simulink model "PID_testing"  (R2023b)
settings: Solver=VariableStepAuto  StartTime=0.0  StopTime=10.0  RelTol=1e-3
values from neighbouring files (symbols this model uses):
  B = 1.36e-6    (= 1.36e-06)    [Admittance_code.m]    (also in motor_model_state_space.m = [0 ; 0 ; 1/L])
  J = 1.62e-6    (= 1.62e-06)    [Admittance_code.m]    (also in motor_model_state_space.m = 1e-06)
  Ke = 0.011    [Admittance_code.m]    (also in motor_model_state_space.m)
  Kt = 0.011    [Admittance_code.m]    (also in motor_model_state_space.m)
  L = 0.58E-3    (= 0.00058)    [Admittance_code.m]    (also in motor_model_state_space.m)
  R = 1.17    [Admittance_code.m]    (also in motor_model_state_space.m)
libraries: slpidlib x1
settings Model: Creator=sayeh  LastModifiedBy=sayeholoumi

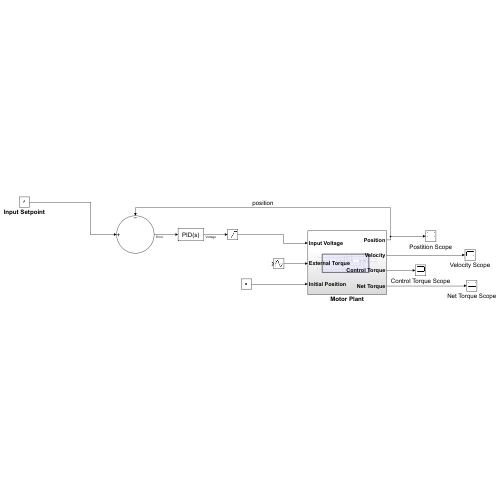
[thumbnail: Simulink's stored preview of the top-level diagram]
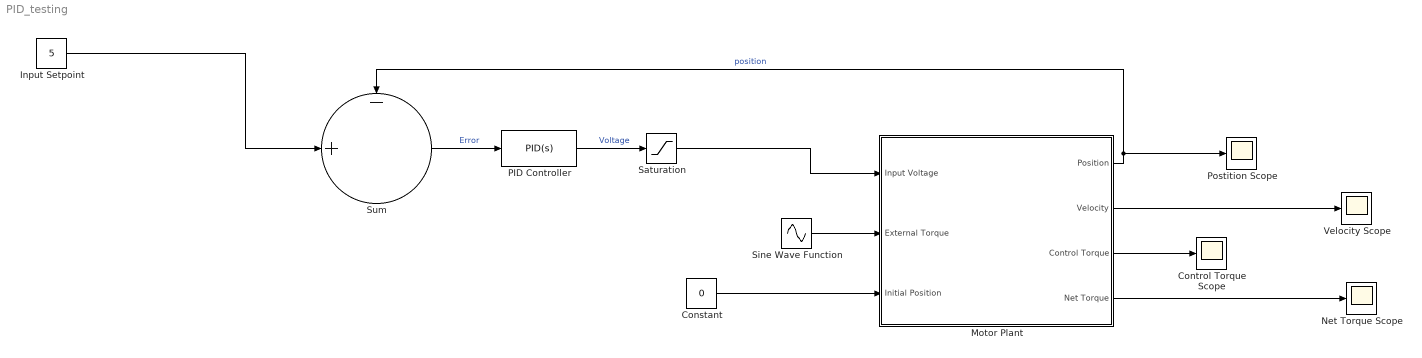
== system PID_testing ==
  Constant : Constant  Value=0
  Control Torque Scope : Scope
  Input Setpoint : Constant  Value=5
  Motor Plant : Subsystem
  Net Torque Scope : Scope
  PID Controller : slpidlib/PID Controller  Controller=PID  Form=Parallel  TimeDomain=Continuous-time  UseExternalTs=off  SampleTime=-1  IntegratorMethod=Forward Euler  FilterMethod=Forward Euler  ControllerParametersSource=internal  P=2  I=10  UseKiTs=off  D=0.0208927627785181  N=1000  UseFilter=on  TunerSelectOption=Transfer Function Based (PID Tuner App)  InitialConditionSource=internal  InitialConditionForIntegrator=0  InitialConditionForFilter=0  DifferentiatorICPrevScaledInput=0  ExternalReset=none  TrackingMode=off  Kt=1  LimitOutput=off  SatLimitsSource=internal  UpperSaturationLimit=inf  LowerSaturationLimit=-inf  LinearizeAsGain=on  AntiWindupMode=none  Kb=1  LimitIntegrator=off  UpperIntegratorSaturationLimit=inf  LowerIntegratorSaturationLimit=-inf  POutMin=[]  POutMax=[]  IOutMin=[]  IOutMax=[]  DOutMin=[]  DOutMax=[]  NOutMin=[]  NOutMax=[]  SumOutMin=[]  SumOutMax=[]  SaturationOutMin=[]  SaturationOutMax=[]  PParamMin=[]  PParamMax=[]  IParamMin=[]  IParamMax=[]  DParamMin=[]  DParamMax=[]  NParamMin=[]  NParamMax=[]  KbParamMin=[]  KbParamMax=[]  KtParamMin=[]  KtParamMax=[]  KbOutMin=[]  KbOutMax=[]  KtOutMin=[]  KtOutMax=[]  IntegratorOutMin=[]  IntegratorOutMax=[]  FilterOutMin=[]  FilterOutMax=[]  SumI1OutMin=[]  SumI1OutMax=[]  SumI2OutMin=[]  SumI2OutMax=[]  SumI3OutMin=[]  SumI3OutMax=[]  SumI4OutMin=[]  SumI4OutMax=[]  SumDOutMin=[]  SumDOutMax=[]  DifferentiatorOutMin=[]  DifferentiatorOutMax=[]  FilterDiffOutCoefMin=[]  FilterDiffOutCoefMax=[]  ReciprocalOutMin=[]  ReciprocalOutMax=[]  SumDenOutMin=[]  SumDenOutMax=[]  SumNumOutMin=[]  SumNumOutMax=[]  DivideOutMin=[]  DivideOutMax=[]  UdiffTsProdOutMin=[]  UdiffTsProdOutMax=[]  NTsProdOutMin=[]  NTsProdOutMax=[]  UintegralTsProdOutMin=[]  UintegralTsProdOutMax=[]  UngainTsProdOutMin=[]  UngainTsProdOutMax=[]  ClampingZeroOutDataTypeStr=Inherit: Inherit via back propagation  ClampingZeroOutMin=[]  ClampingZeroOutMax=[]  FilterDenConstantOutDataTypeStr=Inherit: Inherit via back propagation  FilterDenConstantOutMin=[]  FilterDenConstantOutMax=[]  PCopyOutDataTypeStr=Inherit: Inherit via back propagation  PCopyOutMin=[]  PCopyOutMax=[]  NCopyOutDataTypeStr=Inherit: Inherit via back propagation  NCopyOutMin=[]  NCopyOutMax=[]  IntegratorContinuousStateAttributes=''  IntegratorStateMustResolveToSignalObject=off  IntegratorRTWStateStorageClass=Auto  FilterContinuousStateAttributes=''  FilterStateMustResolveToSignalObject=off  FilterRTWStateStorageClass=Auto  ParallelPVariant=InternalParameters  IdealPVariant=Disabled  IVariant=InternalParameters  DVariant=InternalParameters  IntegratorVariant=Continuous  SatVariant=Disabled  AWVariant=Passthrough  PCopyVariant=Disabled  TRVariant=Disabled  FdbkBlocksVariant=Forward  IdealPFdbkVariant=Disabled  SatFdbkVariant=Disabled  DerivativeFilterVariant=ContFilter  NVariant=InternalParameters  NCopyVariant=Disabled  FilterICVariant=InternalICsFilter  IntegratorICVariant=InternalICs  ExternalResetVariant=Disabled  TRSumVariant=Passthrough  SumFdbkVariant=Disabled  SumVariant=Sum_PID  TsampFilterVariant=InternalTs  TsampNgainVariant=Passthrough  TsampIntegralVariant=Disabled_SignalSpec  ExternalSaturationOutDataTypeStr=Inherit: Same as second input
  Postition Scope : Scope
  Saturation : Saturate  UpperLimit=12  LowerLimit=-12
  Sine Wave Function : Sin  TimeSource=Use external signal  SampleTime=0
  Sum : Sum  Inputs=-+|
  Velocity Scope : Scope
  wires:
  Motor Plant/4(Net Torque) -> Net Torque Scope/1
  Motor Plant/2(Velocity) -> Velocity Scope/1
  Saturation/1 -> Motor Plant/1(Input Voltage)
  Constant/1 -> Motor Plant/3(Initial Position)
  Motor Plant/3(Control Torque) -> Control Torque Scope/1
  Input Setpoint/1 -> Sum/2
  Sine Wave Function/1 -> Motor Plant/2(External Torque)
  Motor Plant/1(Position) -> Postition Scope/1, Sum/1  "position"
  Sum/1 -> PID Controller/1  "Error"
  PID Controller/1 -> Saturation/1  "Voltage"

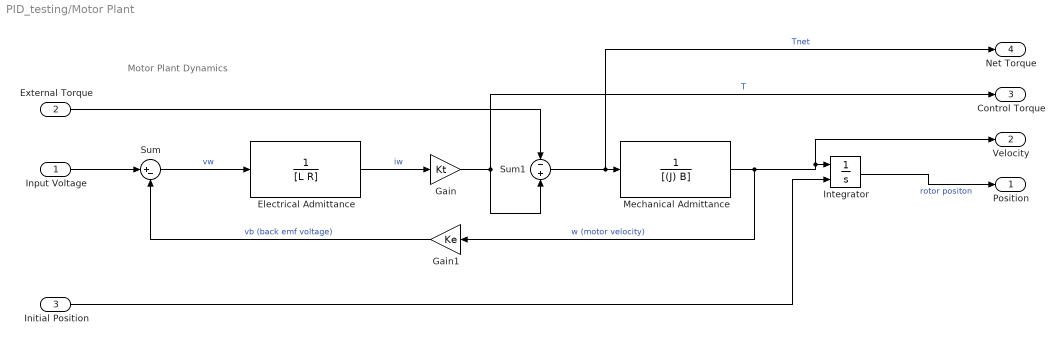
== system PID_testing/Motor Plant ==
  note: Motor Plant Dynamics
  Input Voltage : Inport
  External Torque : Inport  Port=2
  Initial Position : Inport  Port=3
  Electrical Admittance : TransferFcn  Denominator=[L R]
  Gain : Gain  Gain=Kt
  Gain1 : Gain  Gain=Ke
  Integrator : Integrator  InitialConditionSource=external
  Mechanical Admittance : TransferFcn  Denominator=[(J) B]
  Sum : Sum  Inputs=|+-
  Sum1 : Sum  Inputs=-+
  Position : Outport
  Velocity : Outport  Port=2
  Control Torque : Outport  Port=3
  Net Torque : Outport  Port=4
  wires:
  Input Voltage/1 -> Sum/1
  Mechanical Admittance/1 -> Velocity/1, Integrator/1, Gain1/1  "w (motor velocity)"
  Gain1/1 -> Sum/2  "vb (back emf voltage)"
  Integrator/1 -> Position/1  "rotor positon"
  Gain/1 -> Control Torque/1, Sum1/2  "T"
  Electrical Admittance/1 -> Gain/1  "iw"
  Sum/1 -> Electrical Admittance/1  "vw"
  Sum1/1 -> Net Torque/1, Mechanical Admittance/1  "Tnet"
  External Torque/1 -> Sum1/1
  Initial Position/1 -> Integrator/2
